simulink model "sim_main_pqr"  (R2014b)
settings: Solver=ode45  StartTime=0.0  StopTime=tof  FixedStep=dtSim  RelTol=1e-3
values from neighbouring files (symbols this model uses):
  a = -1    [main_pqr.m]    (also in plotlab.m = uint8(a))
  alpha = 1    [main_pqr.m]    (also in main_x12px2.m = -1)
  Ar = -5    [main_pqr.m]    (also in main_x12px2.m = Arv(i))
  Arm1 = Arm1 + [0 a*max(abs(rData(:,3))) ; b*max(abs(rData(:,3))) 0]    [main_pqr.m]    (also in main_x12px2.m = -2)
  b = 1    [main_pqr.m]    (also in plotlab.m = uint8([)
  c = -1    [main_pqr.m]    (also in plotlab.m = get(hLine(i),'color'))
  dtController = dtSim    (= 0.01)    [main_pqr.m]    (also in main_x12px2.m = 0.001)
  epsilon = 0.1    [main_pqr.m]    (also in main_x12px2.m)
  intLimit = 10    [main_pqr.m]    (also in main_x12px2.m)
  K2 = -2    [main_pqr.m]    (also in main_x12px2.m = -10)
  r0 = [0 0]'    [main_pqr.m]    (also in main_x12px2.m = 0)
  rmax = 10000    [main_pqr.m]    (also in main_x12px2.m)
  rmin = -rmax    (= -10000)    [main_pqr.m]    (also in main_x12px2.m)
  x0 = 1*x0    [main_pqr.m]    (also in main_x12px2.m = 10*x0)
settings Model: Creator=Alp  LastModifiedBy=alpmarangoz
settings SolverCC: AutoInsertRateTranBlk=on
settings DataIOCC: SignalLoggingSaveFormat=ModelDataLogs
settings OptimizationCC: ExpressionDepthLimit=2147483647
settings DebuggingCC: UnderspecifiedInitializationDetection=Classic  MergeDetectMultiDrivingBlocksExec=none  FcnCallInpInsideContextMsg=UseLocalSettings  StateNameClashWarn=warning
settings GRTTargetCC: CombineOutputUpdateFcns=off  GRTInterface=on

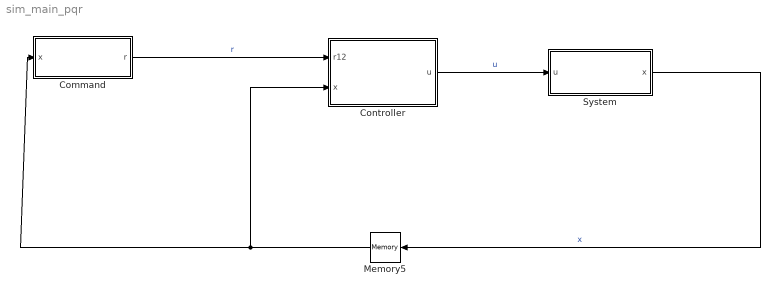
== system sim_main_pqr ==
  Command : Subsystem  TreatAsAtomicUnit=on  SystemSampleTime=dtController
  Controller : Subsystem  TreatAsAtomicUnit=on  SystemSampleTime=dtController
  Memory5 : Memory  X0=x0  InheritSampleTime=on  LinearizeMemory=on  LinearizeAsDelay=on
  System : Subsystem  TreatAsAtomicUnit=on
  wires:
  Command/1(r) -> Controller/1(r12)  "r"
  Controller/1(u) -> System/1(u)  "u"
  System/1(x) -> Memory5/1  "x"
  Memory5/1 -> Controller/2(x), Command/1(x)

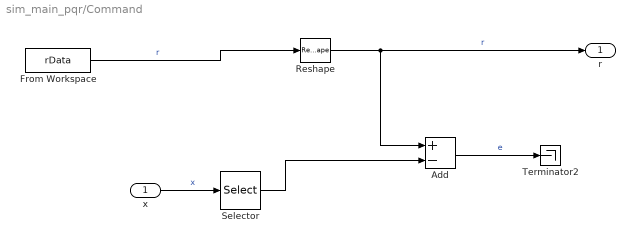
== system sim_main_pqr/Command ==
  x : Inport
  Add : Sum  Inputs=+-
  From Workspace : FromWorkspace  VariableName=rData  OutputAfterFinalValue=Setting to zero
  Reshape : Reshape  OutputDimensionality=Column vector (2-D)
  Selector : Selector  NumberOfDimensions=2  InputPortWidth=3  IndexOptions=Index vector (dialog),Index vector (dialog)  Indices=3,1  OutputSizes=1,1
  Terminator2 : Terminator
  r : Outport
  wires:
  From Workspace/1 -> Reshape/1  "r"
  Reshape/1 -> r/1, Add/1  "r"
  x/1 -> Selector/1  "x"
  Add/1 -> Terminator2/1  "e"
  Selector/1 -> Add/2

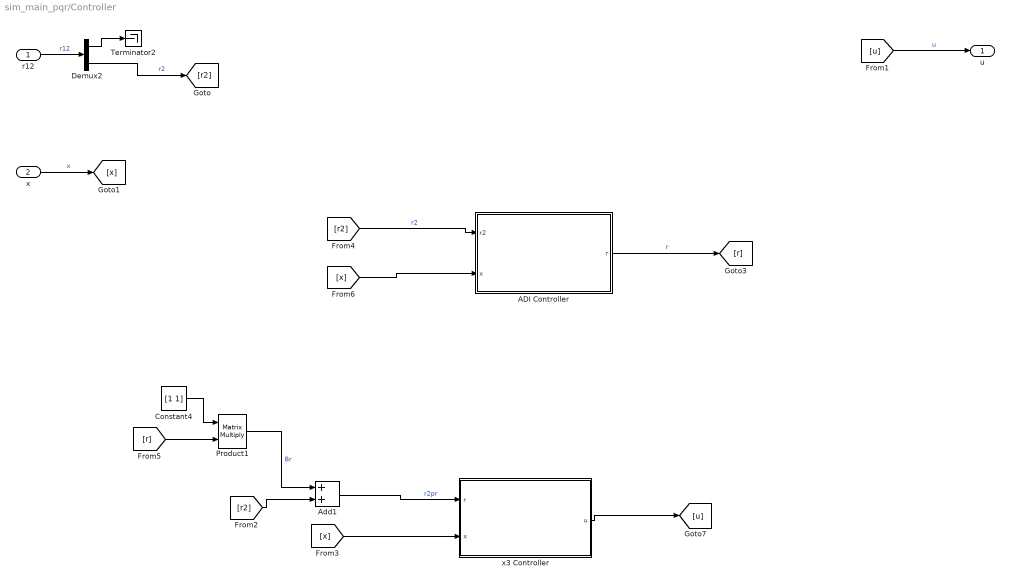
== system sim_main_pqr/Controller ==
  r12 : Inport
  x : Inport  Port=2
  ADI Controller : Subsystem  TreatAsAtomicUnit=on
  Add1 : Sum
  Constant4 : Constant  Value=[1 1]  VectorParams1D=off
  Demux2 : Demux  Outputs=2
  Product1 : Product  Multiplication=Matrix(*)
  Terminator2 : Terminator
  x3 Controller : Subsystem  TreatAsAtomicUnit=on
  u : Outport
  wires:
  [u] -> u/1  "u"
  Demux2/2 -> [r2]  "r2"
  Demux2/1 -> Terminator2/1
  r12/1 -> Demux2/1  "r12"
  ADI Controller/1(r) -> [r]  "r"
  [r2] -> Add1/2
  Add1/1 -> x3 Controller/1(r)  "r2pr"
  [r2] -> ADI Controller/1(r2)  "r2"
  [x] -> ADI Controller/2(x)
  x3 Controller/1(u) -> [u]
  x/1 -> [x]  "x"
  [x] -> x3 Controller/2(x)
  Constant4/1 -> Product1/1
  [r] -> Product1/2
  Product1/1 -> Add1/1  "Br"

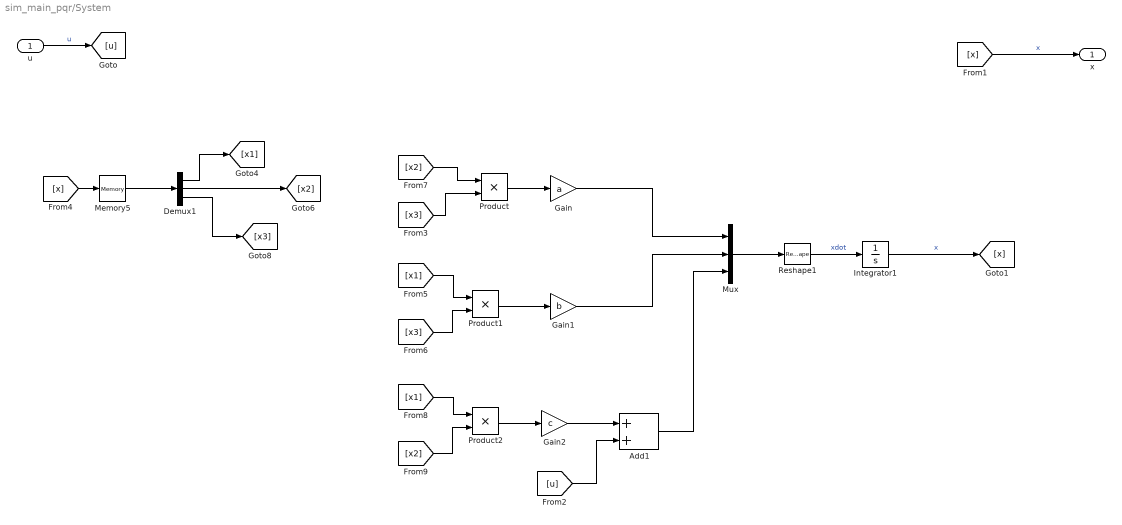
== system sim_main_pqr/System ==
  u : Inport
  Add1 : Sum
  Demux1 : Demux  Outputs=3
  Gain : Gain  Gain=a
  Gain1 : Gain  Gain=b
  Gain2 : Gain  Gain=c
  Integrator1 : Integrator  InitialCondition=x0  LimitOutput=on  UpperSaturationLimit=intLimit  LowerSaturationLimit=-intLimit
  Memory5 : Memory  X0=x0  InheritSampleTime=on  LinearizeMemory=on  LinearizeAsDelay=on
  Mux : Mux  Inputs=3
  Product : Product
  Product1 : Product
  Product2 : Product
  Reshape1 : Reshape  OutputDimensionality=Column vector (2-D)
  x : Outport
  wires:
  u/1 -> [u]  "u"
  [x] -> x/1  "x"
  Reshape1/1 -> Integrator1/1  "xdot"
  Integrator1/1 -> [x]  "x"
  Mux/1 -> Reshape1/1
  Demux1/2 -> [x2]
  Demux1/1 -> [x1]
  Demux1/3 -> [x3]
  [x] -> Memory5/1
  Memory5/1 -> Demux1/1
  [x2] -> Product/1
  [x3] -> Product/2
  Product/1 -> Gain/1
  Product1/1 -> Gain1/1
  Product2/1 -> Gain2/1
  [x3] -> Product1/2
  [x1] -> Product1/1
  [x1] -> Product2/1
  [x2] -> Product2/2
  Gain2/1 -> Add1/1
  [u] -> Add1/2
  Gain/1 -> Mux/1
  Gain1/1 -> Mux/2
  Add1/1 -> Mux/3

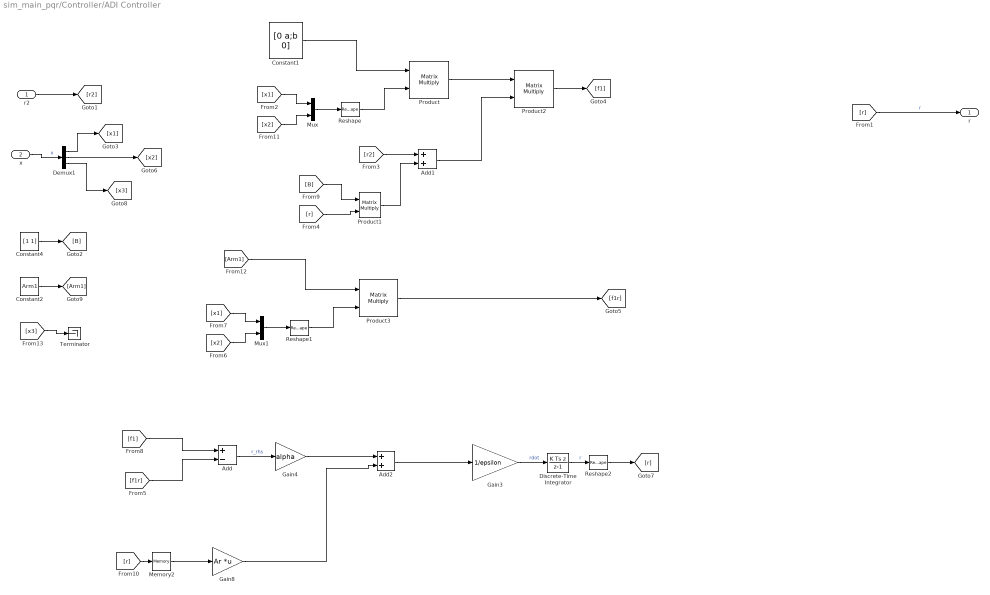
== system sim_main_pqr/Controller/ADI Controller ==
  r2 : Inport
  x : Inport  Port=2
  Add : Sum  Inputs=+-
  Add1 : Sum
  Add2 : Sum
  Constant1 : Constant  Value=[0 a;b 0]  VectorParams1D=off
  Constant2 : Constant  Value=Arm1  VectorParams1D=off
  Constant4 : Constant  Value=[1 1]  VectorParams1D=off
  Demux1 : Demux  Outputs=3
  Discrete-Time Integrator : DiscreteIntegrator  IntegratorMethod=Integration: Backward Euler  InitialCondition=r0  InitialConditionSetting=State (most efficient)  SampleTime=-1  LimitOutput=on  UpperSaturationLimit=rmax  LowerSaturationLimit=rmin
  Gain3 : Gain  Gain=1/epsilon
  Gain4 : Gain  Gain=alpha
  Gain8 : Gain  Gain=Ar  Multiplication=Matrix(K*u)
  Memory2 : Memory  X0=r0  InheritSampleTime=on  LinearizeMemory=on  LinearizeAsDelay=on
  Mux : Mux  Inputs=2
  Mux1 : Mux  Inputs=2
  Product{,1..3} (4 alike) : Product  Multiplication=Matrix(*)
  Reshape : Reshape  OutputDimensionality=Column vector (2-D)
  Reshape1 : Reshape  OutputDimensionality=Column vector (2-D)
  Reshape2 : Reshape  OutputDimensionality=Column vector (2-D)
  Terminator : Terminator
  r : Outport
  wires:
  Gain3/1 -> Discrete-Time Integrator/1  "rdot"
  Discrete-Time Integrator/1 -> Reshape2/1  "r"
  r2/1 -> [r2]
  [r] -> r/1  "r"
  Add/1 -> Gain4/1  "r_rhs"
  [f1] -> Add/1
  [f1r] -> Add/2
  Gain4/1 -> Add2/1
  Add2/1 -> Gain3/1
  [r] -> Memory2/1
  Product2/1 -> [f1]
  Memory2/1 -> Gain8/1
  Gain8/1 -> Add2/2
  x/1 -> Demux1/1  "x"
  Demux1/2 -> [x2]
  Demux1/1 -> [x1]
  Demux1/3 -> [x3]
  Constant4/1 -> [B]
  [x1] -> Mux/1
  [x2] -> Mux/2
  Mux/1 -> Reshape/1
  Constant1/1 -> Product/1
  Reshape/1 -> Product/2
  [B] -> Product1/1
  [r] -> Product1/2
  [r2] -> Add1/1
  Product1/1 -> Add1/2
  Product/1 -> Product2/1
  Add1/1 -> Product2/2
  Constant2/1 -> [Arm1]
  [x1] -> Mux1/1
  [x2] -> Mux1/2
  Mux1/1 -> Reshape1/1
  [Arm1] -> Product3/1
  Reshape1/1 -> Product3/2
  [x3] -> Terminator/1
  Reshape2/1 -> [r]
  Product3/1 -> [f1r]

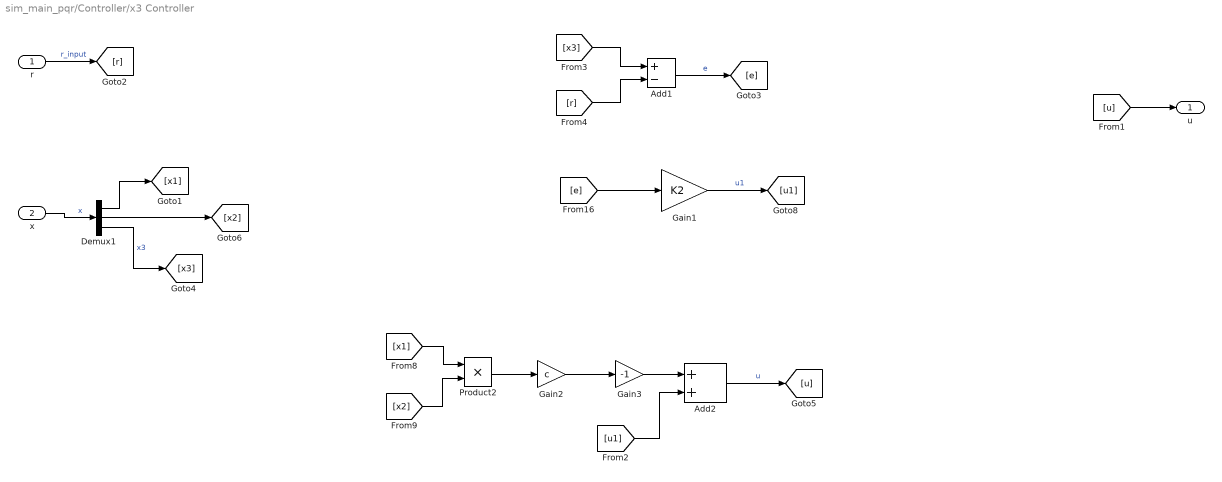
== system sim_main_pqr/Controller/x3 Controller ==
  r : Inport
  x : Inport  Port=2
  Add1 : Sum  Inputs=+-
  Add2 : Sum
  Demux1 : Demux  Outputs=3
  Gain1 : Gain  Gain=K2
  Gain2 : Gain  Gain=c
  Gain3 : Gain  Gain=-1
  Product2 : Product
  u : Outport
  wires:
  [x3] -> Add1/1
  [r] -> Add1/2
  Add1/1 -> [e]  "e"
  r/1 -> [r]  "r_input"
  [u] -> u/1
  [e] -> Gain1/1
  Gain1/1 -> [u1]  "u1"
  x/1 -> Demux1/1  "x"
  Demux1/2 -> [x2]
  Demux1/1 -> [x1]
  Demux1/3 -> [x3]  "x3"
  Product2/1 -> Gain2/1
  [x1] -> Product2/1
  [x2] -> Product2/2
  Gain2/1 -> Gain3/1
  [u1] -> Add2/2
  Add2/1 -> [u]  "u"
  Gain3/1 -> Add2/1
